simulink model "week1_problem1"  (R2020a)
settings: Solver=VariableStepAuto  StartTime=0.0  StopTime=10.0  RelTol=1e-3
model workspace (MAT data in the model file):
  M1 = 100
  M2 = 17.5332429184
  b = 50
  k1 = 50
  k12 = 85.0545304245
settings Model: Creator=hp  LastModifiedBy=hp

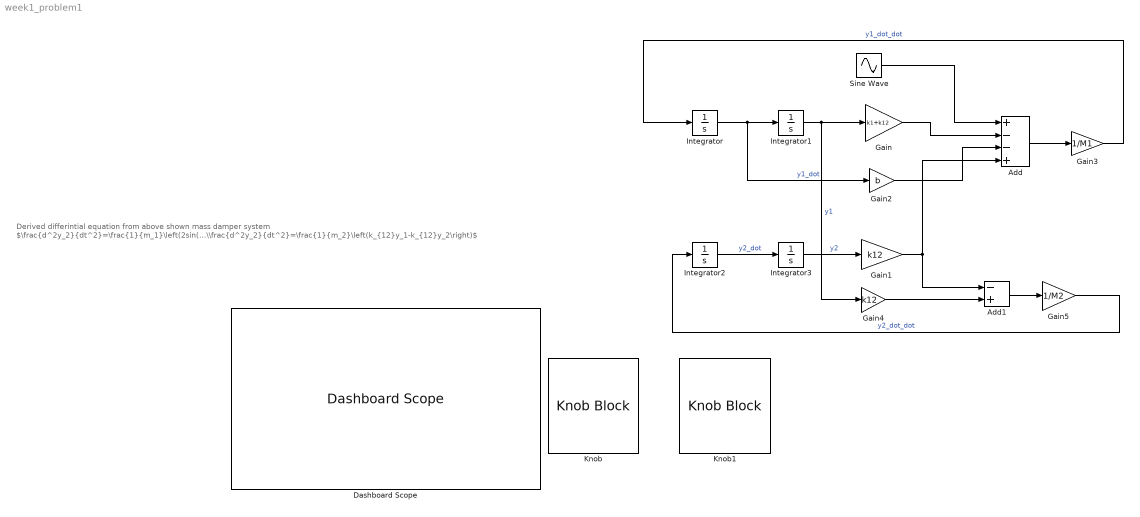
== system week1_problem1 ==
  note: Derived differintial equation from above shown mass damper system
      | $\frac{d^2y_2}{dt^2}=\frac{1}{m_1}\left(2sin(10t)-(k_1+k_2)y_1+k_{12}y_2-b\frac{dy_1}{dt}\right)\\\frac{d^2y_2}{dt^2}=\frac{1}{m_2}\left(k_{12}y_1-k_{12}y_2\right)$
  Add : Sum  Inputs=+--+
  Add1 : Sum  Inputs=-+
  Dashboard Scope : DashboardScope
  Gain : Gain  Gain=k1+k12
  Gain1 : Gain  Gain=k12
  Gain2 : Gain  Gain=b
  Gain3 : Gain  Gain=1/M1
  Gain4 : Gain  Gain=k12
  Gain5 : Gain  Gain=1/M2
  Integrator{,1..3} (4 alike) : Integrator
  Knob : KnobBlock  LabelPosition=Bottom  ScaleMin=1
  Knob1 : KnobBlock  LabelPosition=Bottom  ScaleMin=1
  Sine Wave : Sin  Amplitude=2  Frequency=10  SampleTime=0
  wires:
  Integrator1/1 -> Gain4/1, Gain/1  "y1"
  Integrator2/1 -> Integrator3/1  "y2_dot"
  Integrator/1 -> Gain2/1, Integrator1/1  "y1_dot"
  Gain2/1 -> Add/3
  Gain/1 -> Add/2
  Gain3/1 -> Integrator/1  "y1_dot_dot"
  Integrator3/1 -> Gain1/1  "y2"
  Add/1 -> Gain3/1
  Gain1/1 -> Add1/1, Add/4
  Add1/1 -> Gain5/1
  Gain5/1 -> Integrator2/1  "y2_dot_dot"
  Sine Wave/1 -> Add/1
  Gain4/1 -> Add1/2
